simulink model "gate"  (R2013b)
settings: Solver=ode45  StartTime=0.0  StopTime=10.0  RelTol=1e-3
libraries: xbsIndex_r4 x3, casper_library_misc x1
settings Model: Creator=root  LastModifiedBy=root

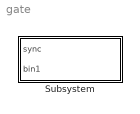
== system gate ==
  Subsystem : Subsystem  mask{bin_len=1, bitwidth=20}
      mask prompts: bin_len "bin length"; bitwidth "bit width"
      mask init:
      | config.source = str2func('init_gate');
      | config.toplevel = gcb;
      | xBlock(config, {bin_len, bitwidth});

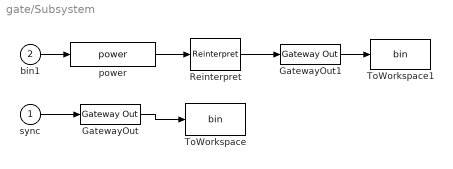
== system gate/Subsystem ==
  sync : Inport
  bin1 : Inport  Port=2
  GatewayOut : xbsIndex_r4/Gateway Out  inherit_from_input=on  hdl_port=on  timing_constraint=None  locs_specified=off  LOCs={}  UseAsDAC=off  DACChannel='1'  block_type=gatewayout
  GatewayOut1 : xbsIndex_r4/Gateway Out  inherit_from_input=on  hdl_port=on  timing_constraint=None  locs_specified=off  LOCs={}  UseAsDAC=off  DACChannel='1'  block_type=gatewayout
  Reinterpret : xbsIndex_r4/Reinterpret  force_arith_type=off  arith_type=Unsigned  force_bin_pt=on  bin_pt=0  block_type=reinterpret
  ToWorkspace : ToWorkspace  VariableName=bin  SampleTime=-1  SaveFormat=Timeseries
  ToWorkspace1 : ToWorkspace  VariableName=bin  SampleTime=-1  SaveFormat=Timeseries
  power : casper_library_misc/power  BitWidth=20  add_latency=2  mult_latency=3
  wires:
  GatewayOut1/1 -> ToWorkspace1/1
  Reinterpret/1 -> GatewayOut1/1
  power/1 -> Reinterpret/1
  bin1/1 -> power/1
  GatewayOut/1 -> ToWorkspace/1
  sync/1 -> GatewayOut/1
